simulink model "Drainingofwater"  (R2021a)
settings: Solver=VariableStepAuto  StartTime=0.0  StopTime=128  RelTol=1e-3
settings Model: Creator=42077  LastModifiedBy=42077

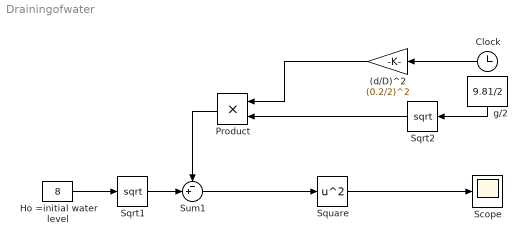
== system Drainingofwater ==
  (d/D)^2 : Gain  Gain=(0.2/2)^2  SaturateOnIntegerOverflow=on  OutDataTypeStr=Inherit: Same as input  ParamDataTypeStr=Inherit: Same as input
  Clock : Clock
  Ho =initial water level : Constant  Value=8
  Product : Product
  Scope : Scope
  Sqrt1 : Sqrt  SaturateOnIntegerOverflow=on
  Sqrt2 : Sqrt  SaturateOnIntegerOverflow=on
  Square : Math  Operator=square  SaturateOnIntegerOverflow=on
  Sum1 : Sum  Inputs=-+|
  g/2 : Constant  Value=9.81/2
  wires:
  Ho =initial water level/1 -> Sqrt1/1
  Sqrt1/1 -> Sum1/2
  (d/D)^2/1 -> Product/1
  Clock/1 -> (d/D)^2/1
  Product/1 -> Sum1/1
  Sum1/1 -> Square/1
  Square/1 -> Scope/1
  Sqrt2/1 -> Product/2
  g/2/1 -> Sqrt2/1
